simulink model "drone_model"  (R2023b)
settings: Solver=VariableStepAuto  StartTime=0.0  StopTime=70  RelTol=1e-3
InitFcn:
  | clc;
  | 
  | I_xx = 228.211;
  | I_yy = 228.211;
  | I_zz = 246.355;
  | 
  | 
  | 
  | m = 327.316; %mass
  | g = 9.81; %gravitational acceleration
  | p = 1.225; %density of the environment
  | 
  | 
  | %aerodynamic forces are negligible
  | C_L = 0;
  | C_D = 0;
  | 
  | 
  | %Vector from center of gravity to the
  | %center of pressure
  | r_CP = [ 0.2; 0.0; 0.0];
  | 
  | k_r = 0.0001; %Aerodynamic damping coefficient
  | 
  | c = 20; %coefficient to calculate counter-moment
  | 
  | l = 2; %Rotor moment arm length
  | 
  | T_max = 1500; %Max thrust
  | 
  | tau = 0.05;
  | 
  | v_B = [0; 0; 0];
  | 
  | w_B = [0; 0; 0];
  | 
  | x_I = [0;0; -5];
  | 
  | euler_angles = [0;0;0];
settings Model: Creator=nijatabbasov  LastModifiedBy=nijatabbasov

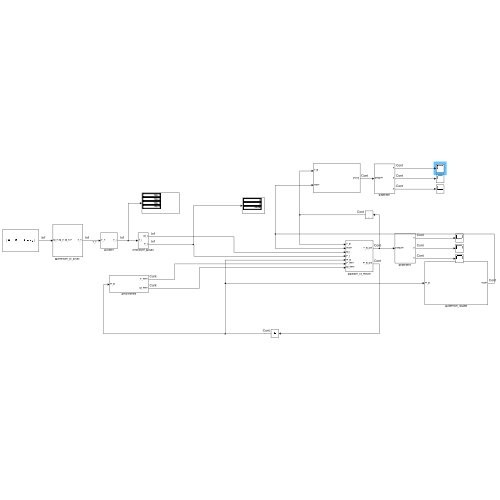
[thumbnail: Simulink's stored preview of the top-level diagram]
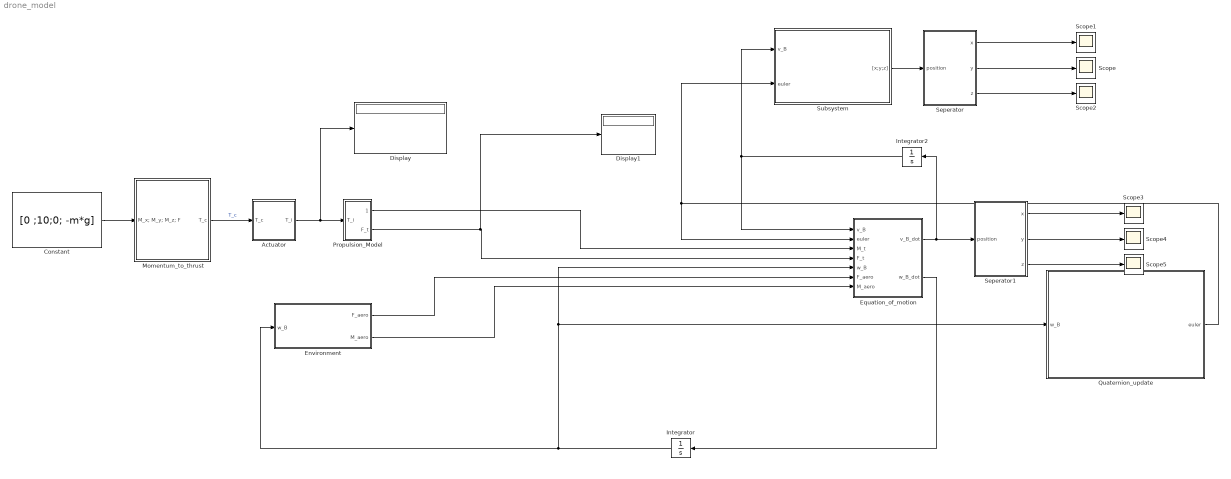
== system drone_model ==
  Actuator : Subsystem
  Constant : Constant  Value=[0 ;10;0; -m*g]
  Display : Display
  Display1 : Display
  Environment : Subsystem
  Equation_of_motion : Subsystem
  Integrator : Integrator  InitialCondition=[0; 0; 0]
  Integrator2 : Integrator  InitialCondition=[0; 0; 0]
  "Momentum_to_thrust " : Subsystem
  Propulsion_Model : Subsystem
  Quaternion_update : Subsystem
  Scope{,1..5} (6 alike) : Scope
  Seperator : Subsystem
  Seperator1 : Subsystem
  Subsystem : Subsystem
  wires:
  Constant/1 -> "Momentum_to_thrust "/1(M_x; M_y; M_z; F)
  Integrator/1 -> Equation_of_motion/5(w_B), Quaternion_update/1(w_B), Environment/1(w_B)
  Integrator2/1 -> Equation_of_motion/1(v_B), Subsystem/1(v_B)
  Propulsion_Model/1(M_t) -> Equation_of_motion/3(M_t)
  Propulsion_Model/2(F_t) -> Display1/1, Equation_of_motion/4(F_t)
  Environment/1(F_aero) -> Equation_of_motion/6(F_aero)
  Environment/2(M_aero) -> Equation_of_motion/7(M_aero)
  "Momentum_to_thrust "/1(T_c) -> Actuator/1(T_c)  "T_c"
  Actuator/1(T_i) -> Display/1, Propulsion_Model/1(T_i)
  Quaternion_update/1(euler) -> Subsystem/2(euler), Equation_of_motion/2(euler)
  Equation_of_motion/2(w_B_dot) -> Integrator/1
  Subsystem/1("[x;y;z]") -> Seperator/1(position)
  Seperator/1(x) -> Scope1/1
  Seperator/2(y) -> Scope/1
  Seperator/3(z) -> Scope2/1
  Seperator1/3(z) -> Scope5/1
  Equation_of_motion/1(v_B_dot) -> Seperator1/1(position), Integrator2/1
  Seperator1/1(x) -> Scope3/1
  Seperator1/2(y) -> Scope4/1

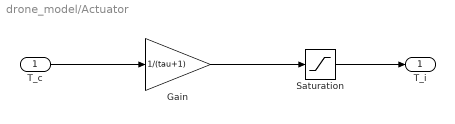
== system drone_model/Actuator ==
  T_c : Inport
  Gain : Gain  Gain=1/(tau+1)
  Saturation : Saturate  UpperLimit=1500  LowerLimit=0
  T_i : Outport
  wires:
  T_c/1 -> Gain/1
  Gain/1 -> Saturation/1
  Saturation/1 -> T_i/1

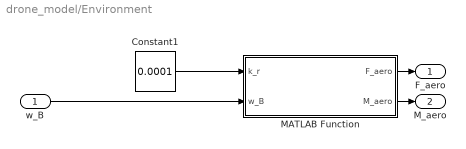
== system drone_model/Environment ==
  w_B : Inport
  Constant1 : Constant  Value=0.0001
  MATLAB Function : MATLAB Function  TreatAsAtomicUnit=on
  F_aero : Outport
  M_aero : Outport  Port=2
  wires:
  w_B/1 -> MATLAB Function/2(w_B)
  MATLAB Function/2(M_aero) -> M_aero/1
  MATLAB Function/1(F_aero) -> F_aero/1
  Constant1/1 -> MATLAB Function/1(k_r)

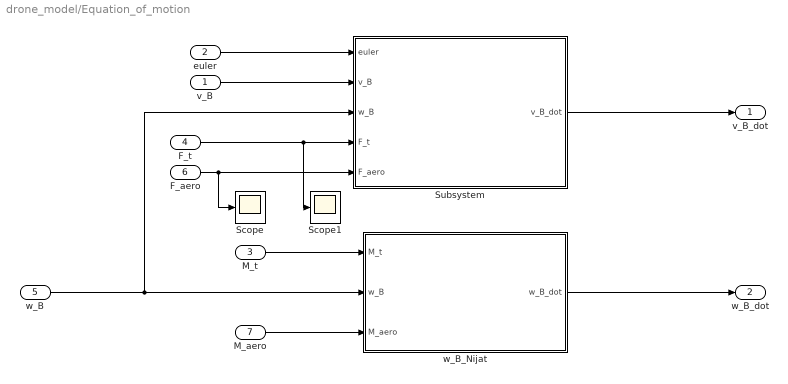
== system drone_model/Equation_of_motion ==
  v_B : Inport
  euler : Inport  Port=2
  M_t : Inport  Port=3
  F_t : Inport  Port=4
  w_B : Inport  Port=5
  F_aero : Inport  Port=6
  M_aero : Inport  Port=7
  Scope : Scope
  Scope1 : Scope
  Subsystem : Subsystem
  w_B_Nijat : Subsystem
  v_B_dot : Outport
  w_B_dot : Outport  Port=2
  wires:
  euler/1 -> Subsystem/1(euler)
  Subsystem/1(v_B_dot) -> v_B_dot/1
  w_B/1 -> Subsystem/3(w_B), w_B_Nijat/2(w_B)
  F_aero/1 -> Subsystem/5(F_aero), Scope/1
  F_t/1 -> Subsystem/4(F_t), Scope1/1
  v_B/1 -> Subsystem/2(v_B)
  M_t/1 -> w_B_Nijat/1(M_t)
  w_B_Nijat/1(w_B_dot) -> w_B_dot/1
  M_aero/1 -> w_B_Nijat/3(M_aero)

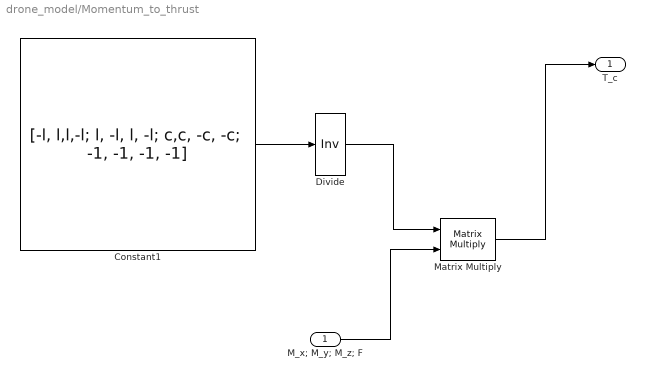
== system drone_model/Momentum_to_thrust  ==
  M_x; M_y; M_z; F : Inport
  Constant1 : Constant  Value=[-l, l,l,-l; l, -l, l, -l; c,c, -c, -c; -1, -1, -1, -1]
  Divide : Product  Inputs=/  Multiplication=Matrix(*)  OutDataTypeStr=double
  Matrix Multiply : Product  Multiplication=Matrix(*)
  T_c : Outport
  wires:
  M_x; M_y; M_z; F/1 -> Matrix Multiply/2
  Matrix Multiply/1 -> T_c/1
  Divide/1 -> Matrix Multiply/1
  Constant1/1 -> Divide/1

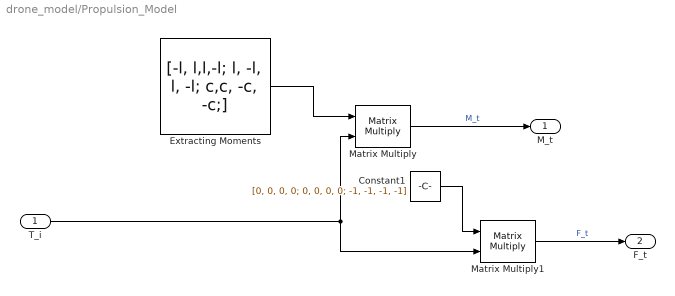
== system drone_model/Propulsion_Model ==
  T_i : Inport
  Constant1 : Constant  Value=[0, 0, 0, 0; 0, 0, 0, 0; -1, -1, -1, -1]
  Extracting Moments : Constant  Value=[-l, l,l,-l; l, -l, l, -l; c,c, -c, -c;]
  Matrix Multiply : Product  Multiplication=Matrix(*)
  Matrix Multiply1 : Product  Multiplication=Matrix(*)
  M_t : Outport
  F_t : Outport  Port=2
  wires:
  T_i/1 -> Matrix Multiply1/2, Matrix Multiply/2
  Matrix Multiply/1 -> M_t/1  "M_t"
  Extracting Moments/1 -> Matrix Multiply/1
  Matrix Multiply1/1 -> F_t/1  "F_t"
  Constant1/1 -> Matrix Multiply1/1

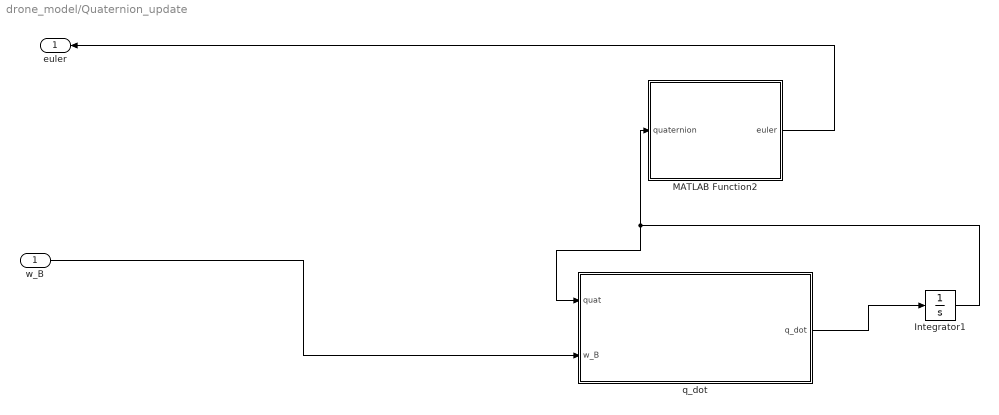
== system drone_model/Quaternion_update ==
  w_B : Inport
  Integrator1 : Integrator  InitialCondition=[1; 0; 0; 0]
  MATLAB Function2 : MATLAB Function  TreatAsAtomicUnit=on
  q_dot : MATLAB Function  TreatAsAtomicUnit=on
  euler : Outport
  wires:
  MATLAB Function2/1(euler) -> euler/1
  w_B/1 -> q_dot/2(w_B)
  Integrator1/1 -> MATLAB Function2/1(quaternion), q_dot/1(quat)
  q_dot/1(q_dot) -> Integrator1/1

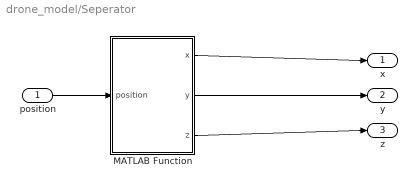
== system drone_model/Seperator ==
  position : Inport
  MATLAB Function : MATLAB Function  TreatAsAtomicUnit=on
  x : Outport
  y : Outport  Port=2
  z : Outport  Port=3
  wires:
  MATLAB Function/2(y) -> y/1
  position/1 -> MATLAB Function/1(position)
  MATLAB Function/1(x) -> x/1
  MATLAB Function/3(z) -> z/1

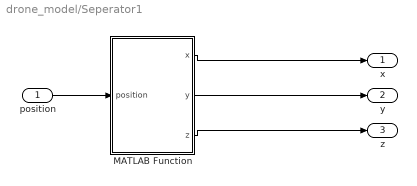
== system drone_model/Seperator1 ==
  position : Inport
  MATLAB Function : MATLAB Function  TreatAsAtomicUnit=on
  x : Outport
  y : Outport  Port=2
  z : Outport  Port=3
  wires:
  MATLAB Function/2(y) -> y/1
  position/1 -> MATLAB Function/1(position)
  MATLAB Function/1(x) -> x/1
  MATLAB Function/3(z) -> z/1

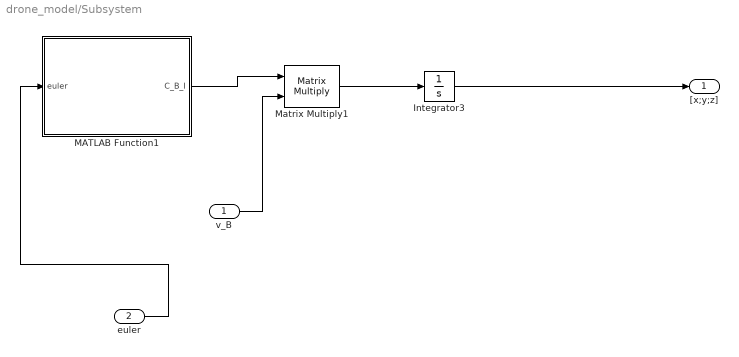
== system drone_model/Subsystem ==
  v_B : Inport
  euler : Inport  Port=2
  Integrator3 : Integrator  InitialCondition=[0; 0; -5]
  MATLAB Function1 : MATLAB Function  TreatAsAtomicUnit=on
  Matrix Multiply1 : Product  Multiplication=Matrix(*)
  "[x;y;z]" : Outport
  wires:
  v_B/1 -> Matrix Multiply1/2
  euler/1 -> MATLAB Function1/1(euler)
  Integrator3/1 -> "[x;y;z]"/1
  MATLAB Function1/1(C_B_I) -> Matrix Multiply1/1
  Matrix Multiply1/1 -> Integrator3/1

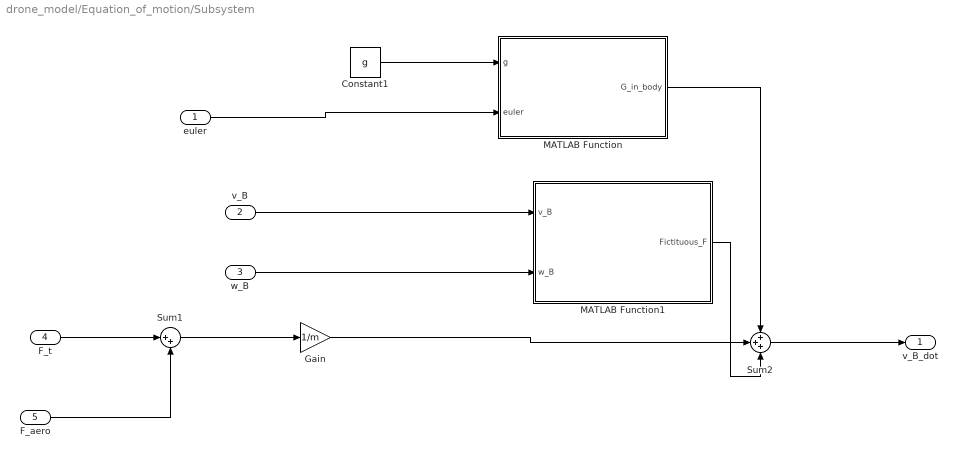
== system drone_model/Equation_of_motion/Subsystem ==
  euler : Inport
  v_B : Inport  Port=2
  w_B : Inport  Port=3
  F_t : Inport  Port=4
  F_aero : Inport  Port=5
  Constant1 : Constant  Value=g
  Gain : Gain  Gain=1/m
  MATLAB Function : MATLAB Function  TreatAsAtomicUnit=on
  MATLAB Function1 : MATLAB Function  TreatAsAtomicUnit=on
  Sum1 : Sum  Inputs=|++
  Sum2 : Sum  Inputs=+++
  v_B_dot : Outport
  wires:
  F_t/1 -> Sum1/1
  F_aero/1 -> Sum1/2
  w_B/1 -> MATLAB Function1/2(w_B)
  MATLAB Function/1(G_in_body) -> Sum2/1
  Constant1/1 -> MATLAB Function/1(g)
  euler/1 -> MATLAB Function/2(euler)
  MATLAB Function1/1(Fictituous_F) -> Sum2/3
  Gain/1 -> Sum2/2
  v_B/1 -> MATLAB Function1/1(v_B)
  Sum2/1 -> v_B_dot/1
  Sum1/1 -> Gain/1

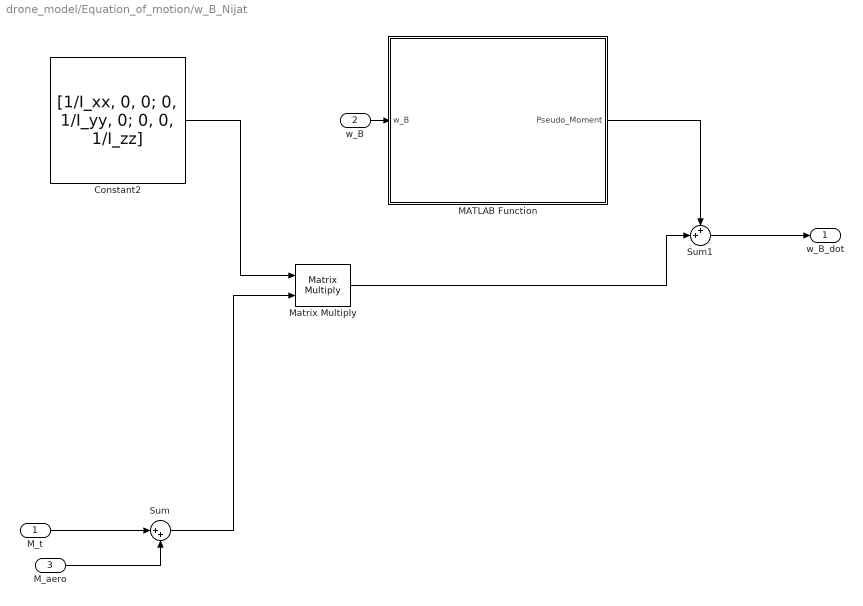
== system drone_model/Equation_of_motion/w_B_Nijat ==
  M_t : Inport
  w_B : Inport  Port=2
  M_aero : Inport  Port=3
  Constant2 : Constant  Value=[1/I_xx, 0, 0; 0, 1/I_yy, 0; 0, 0, 1/I_zz]
  MATLAB Function : MATLAB Function  TreatAsAtomicUnit=on
  Matrix Multiply : Product  Multiplication=Matrix(*)
  Sum : Sum  Inputs=|++
  Sum1 : Sum  Inputs=++|
  w_B_dot : Outport
  wires:
  M_t/1 -> Sum/1
  Matrix Multiply/1 -> Sum1/2
  w_B/1 -> MATLAB Function/1(w_B)
  Sum1/1 -> w_B_dot/1
  M_aero/1 -> Sum/2
  MATLAB Function/1(Pseudo_Moment) -> Sum1/1
  Constant2/1 -> Matrix Multiply/1
  Sum/1 -> Matrix Multiply/2

== matlab function drone_model/Equation_of_motion/Subsystem/MATLAB Function ==
  data: g input; G_in_body output; euler input
function G_in_body = G_in_body(g, euler)
    % This function evaluates derivative of vehicle speed in body frame 
    % and angular velocity of the center of gravity of the vehicle
    %Acceler is (F_thrust + F_aero)/m
    phi = euler(1);
    theta = euler(2);
    

    
    frame_change = [-sin(theta); sin(phi)*cos(theta); cos(phi)* cos(theta)];


    G_in_body = frame_change * g;
   
end

== matlab function drone_model/Environment/MATLAB Function ==
  data: k_r input; F_aero output; w_B input; M_aero output
function [F_aero, M_aero] = F_aero_M_aero(k_r, w_B)

    F_aero = 0;
    M_aero = - k_r * w_B;

== matlab function drone_model/Equation_of_motion/Subsystem/MATLAB Function1 ==
  data: v_B input; Fictituous_F output; w_B input
function Fictituous_F = Fictituous_F(v_B, w_B)
    % This function evaluates derivative of vehicle speed in body frame 
    % and angular velocity of the center of gravity of the vehicle
    
    p = w_B(1);
    q = w_B(2);
    r = w_B(3);


    w_x = [0, -r,  q;
           r,  0, -p;
          -1   p   0   ];

   

    Fictituous_F = w_x * v_B;
    
end

== matlab function drone_model/Equation_of_motion/w_B_Nijat/MATLAB Function ==
  data: w_B input; Pseudo_Moment output
function Pseudo_Moment = Pseudo_Moment(w_B)
    % This function evaluates value of w*(Iw)
   
    p = w_B(1);
    q = w_B(2);
    r = w_B(3);


    
    
   
    I_xx = 228.211; 
    I_yy = 228.211;
    I_zz = 246.355;



    Pseudo_Moment = [(I_yy-I_zz)*q*r/I_xx; (I_zz - I_xx)*p*r/I_yy; (I_xx - I_yy)*p*q/I_zz];
   
    
end

== matlab function drone_model/Quaternion_update/q_dot ==
  data: quat input; q_dot output; w_B input
function q_dot = q_dot(quat, w_B)
    q_0 = quat(1);
    q_1 = quat(2);
    q_2 = quat(3);
    q_3 = quat(4);

    p = w_B(1);
    q = w_B(2);
    r = w_B(3);

    epsilon_q = 1-(q_0^2 + q_1^2 + q_2^2 + q_3^2);

    C_k = 5;
    A = [0, -p, -q, -r;
         p,  0,  r, -q;
         q, -r,  0,  p;
         r,  q, -p,  0];

    
    q_dot = 1/2 * A *quat  + C_k * epsilon_q*quat;


end

== matlab function drone_model/Seperator/MATLAB Function ==
  data: x output; position input; y output; z output
function [x,y,z] = fcn(position)
    x = position(1);
    y = position(2);
    z = position(3);
    
    
end

== matlab function drone_model/Seperator1/MATLAB Function ==
  data: x output; position input; y output; z output
function [x,y,z] = fcn(position)
    x = position(1);
    y = position(2);
    z = position(3);
    
    
end

== matlab function drone_model/Subsystem/MATLAB Function1 ==
  data: euler input; C_B_I output
function C_B_I = C_B_I(euler)
    phi = euler(1);
    theta = euler(2);
    psi = euler(3);

    C_I_B = [cos(theta)*cos(psi),  cos(theta)*sin(psi), -sin(theta);
        sin(phi)*sin(theta)*cos(psi)-cos(phi)*sin(psi), sin(phi)*sin(theta)*sin(psi) + cos(phi)*cos(psi), sin(phi)*cos(theta);
        cos(phi)*sin(theta)*cos(psi) + sin(phi)*sin(psi), cos(phi)*sin(theta)*sin(psi) - sin(phi)*cos(psi), cos(phi)*cos(theta)];
    C_B_I = transpose(C_I_B);

== matlab function drone_model/Quaternion_update/MATLAB Function2 ==
  data: quaternion input; euler output
function euler = quaternionToEuler(quaternion)
    % quaternionToEuler converts a quaternion to Euler angles (roll, pitch, yaw).
    q_0 = quaternion(1);
    q_1 = quaternion(2);
    q_2 = quaternion(3);
    q_3 = quaternion(4);

    c_11 = q_0^2 + q_1^2 - q_2^2 - q_3^2;
    c_12 = 2*(q_1*q_2 + q_0*q_3);
    c_13 = 2*(q_1 * q_3 - q_0 *q_2);
    c_23 = 2*(q_2 * q_3 + q_0 * q_1);
    c_33 = q_0^2 + q_3^2 - q_1^2 - q_2^2;


    phi = atan(c_23/ c_33);
    theta = asin(-c_13);
    psi = atan(c_12/c_11);

    euler = [phi; theta; psi];
